simulink model "MotorControlLibNEWFixedP_FULL"  (R2020b)
settings: Solver=FixedStepDiscrete  StartTime=0.0  StopTime=100  FixedStep=Ts  RelTol=1e-3
values from neighbouring files (symbols this model uses):
  Ki_Iab_EMFobs = 1600.0    [MotorControl.sldd]
  Kp_Iab_EMFobs = 0.255    [MotorControl.sldd]
  p = 8/2    (= 4)    [MotorControlLibData.m]    (also in local_pmsm_torque_control_data.m = 8)
  Ts = 250.0e-06    (= 0.00025)    [MotorControlLibData.m]    (also in local_pmsm_torque_control_data.m = 5e-06)
undefined symbols (not defined in the file or in its folder): BrkPoints, CuttOffFreq_c, d_q_Voltage_Limiter_sat_neg, d_q_Voltage_Limiter_sat_pos, DiscIntNeverNeededParam, Down, dSoll, EMFobsLdGain, EMFobsRS, Ki_dAxis, Ki_qAxis, Kp_dAxis, Kp_qAxis, MaxBckEMFVol_sat_neg, MaxBckEMFVol_sat_pos, NumBits1, NumBits2, qSoll, Slope1, Slope2, TqToIqConst, TsIntern, Up
libraries: simulink x12, pid_lib x4, eePwmGenerator x3, simulink_extras x2
(part 1 of 2)
settings Model: DataDictionary=MotorControl.sldd  NumberOfSteps=50  Creator=unix  LastModifiedBy=unix
settings SolverCC: AutoInsertRateTranBlk=on
settings DebuggingCC: ArrayBoundsChecking=warning  SignalInfNanChecking=warning  SignalRangeChecking=warning  CheckMatrixSingularityMsg=warning  ParameterOverflowMsg=warning  ParameterUnderflowMsg=warning  ParameterPrecisionLossMsg=none  UnderSpecifiedDataTypeMsg=warning

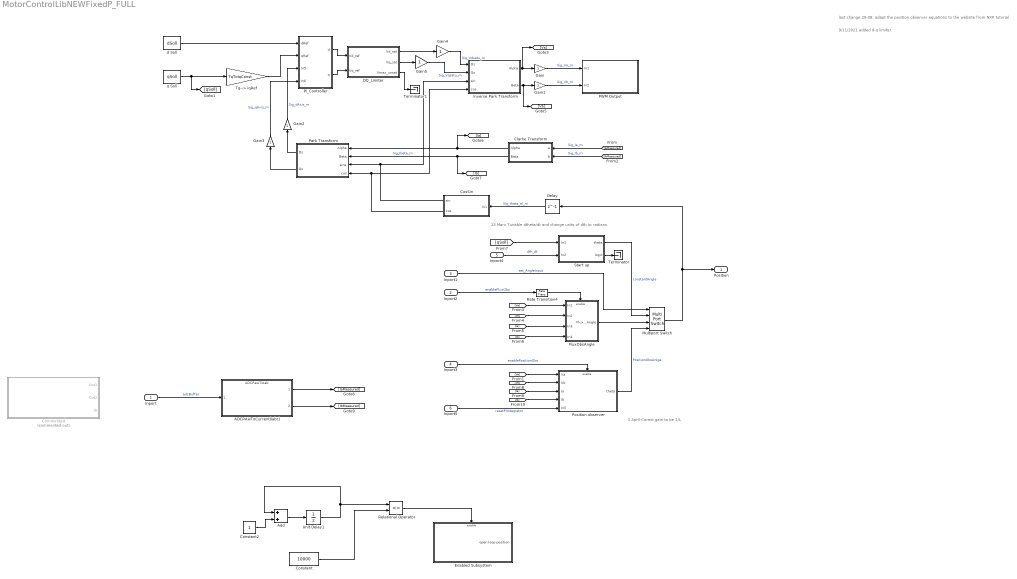
== system MotorControlLibNEWFixedP_FULL ==
  note: 3 April-Corect gain to be 1/L
  note: 9/11/2021 added d-q limiter.
  note: 23 Marz Tunable dtheta/dt and change units of dth to radians
  note: last change 29-08: adapt the position observer equations to the website from NXP tutorial
  Inport : Inport
  Inport2 : Inport  Port=2  OutDataTypeStr=boolean  SampleTime=5*Ts
      settings: AttributesFormatString=%<SampleTime>
  Inport1 : Inport  Port=3  OutDataTypeStr=uint8  SampleTime=5*Ts
      settings: AttributesFormatString=%<SampleTime>
  Inport3 : Inport  Port=4  OutDataTypeStr=boolean  SampleTime=5*Ts
      settings: AttributesFormatString=%<SampleTime>
  Inport4 : Inport  Port=5
  Inport5 : Inport  Port=6  OutDataTypeStr=boolean  SampleTime=5*Ts
      settings: AttributesFormatString=%<SampleTime>
  ADCRAwToCurrent(Iabc) : ModelReference  ModelNameDialog=ADCRawToIab  ModelReferenceVersion=3.2
  Add : Sum  OutDataTypeStr=uint16
  Clarke Transform : Subsystem  VariantControl=Variant2  mask(Clarke Transform){}
      mask help:
      | <p>Compute Clarke transformation on balanced 3-phase inputs into balanced 2-phase orthogonal outputs.
      | <br>
      | <br>
      | The block accepts two signals out of three phases, and outputs corresponding &alpha;-&beta; axis components, where phase-a axis is aligned with alpha axis.</p>
      mask Help: eval('mcb.internal.helpview(''clarketransform'')')
      mask Display: mcb.internal.drawIcons('Clarke',1);
  Commented : Subsystem  Commented=on
  Constant : Constant  Value=10000  OutDataTypeStr=uint16
  Constant2 : Constant  OutDataTypeStr=uint8
  CosSin : Subsystem
  DQ_Limiter : Subsystem  TreatAsAtomicUnit=on  SystemSampleTime=5*Ts  mask(DQ Limiter){Vmax=d_q_Voltage_Limiter_sat_pos}
      mask prompts: Vmax "D-Q saturation limit:"
      mask help:
      | Implement saturation on reference dq voltages, with respect to phase voltage peak limit.
      |
      | The block accepts reference values of d and q axis voltages, and outputs corresponding saturated values along with unsaturated peak value to initiate field weakening control.
      |
      | Enter the phase voltage peak limit in the dialog box to initiate saturation.
      settings: RTWFcnNameOpts=Use subsystem name
      mask Help: eval('mcb.internal.helpview(''dqlimiter'')')
  Delay : Delay  DelayLength=1  SampleTime=5*Ts
      settings: AttributesFormatString=%<SampleTime>
  Enabled Subsystem : Subsystem  TreatAsAtomicUnit=on
  FluxObsAngle : Subsystem
      settings: RTWFcnNameOpts=Use subsystem name
  Gain{,1..3} (4 alike) : Gain  OutDataTypeStr=Inherit: Same as input  ParamDataTypeStr=Inherit: Same as input
  Gain4 : Gain  OutDataTypeStr=Inherit: Inherit via back propagation
  Gain5 : Gain  OutDataTypeStr=Inherit: Inherit via back propagation
  Inverse Park Transform : Subsystem  SystemSampleTime=250*Ts  mask(Inverse Park Transform){AxisAlignment=D-axis}
      mask prompts: AxisAlignment "Alpha (phase-a) axis alignment:"
      mask help:
      | <p>Compute Inverse Park transformation on rotating reference frame inputs into stationary reference frame outputs.
      | <br><br>
      | The block accepts the following:
      | <ul>
      | <li>d-q axis components in rotating reference frame</li>
      | <li>Sine and cosine values of corresponding angle of transformation</li>
      | </ul>
      | The block outputs &alpha;-&beta; axis components in stationary reference frame.
      | <br><br>
      | D-axis alignment with alpha (phase-a) is popular in motor control theory while Q-axis alignment with alpha (phase-a) is more suitable for power conversion applications.</p>
      mask Help: eval('mcb.internal.helpview(''inverseparktransform'')')
      mask TypeOptions AxisAlignment: D-axis | Q-axis
  Multiport Switch : MultiPortSwitch  DataPortOrder=Zero-based contiguous  zeroidx=on
  PI_Controller : Subsystem  TreatAsAtomicUnit=on  SystemSampleTime=5*Ts
      settings: RTWFcnNameOpts=Use subsystem name
  PWM Output : Subsystem
  Park Transform : Subsystem  SystemSampleTime=250*Ts  mask(Park Transform){AxisAlignment=D-axis}
      mask prompts: AxisAlignment "Alpha (phase-a) axis alignment:"
      mask help:
      | <p>Compute Park transformation on stationary reference frame inputs into rotating reference frame outputs.
      | <br><br>
      | The block accepts the following:
      | <ul>
      |   <li>&alpha;-&beta; axis components in stationary reference frame</li>
      |   <li>Sine and cosine values of corresponding angle of transformation</li>
      | </ul>
      | The block outputs direct and quadrature axis components in rotating reference frame.
      | <br><br>
      | D-axis alignment with alpha (phase-a) is popular in motor control theory while Q-axis alignment with alpha (phase-a) is more suitable for power conversion applications.</p>
      mask Help: eval('mcb.internal.helpview(''parktransform'')')
      mask TypeOptions AxisAlignment: D-axis | Q-axis
      mask Display: mcb.internal.drawIcons('Park',1);
  Position observer : Subsystem
  Rate Transition4 : RateTransition
  Relational Operator : RelationalOperator  Operator=<=  OutDataTypeStr=boolean  RndMeth=Simplest
  Start up : Subsystem  TreatAsAtomicUnit=on  SystemSampleTime=5*Ts
  Terminator : Terminator
  Terminator1 : Terminator
  Tq--> iqRef : Gain  Gain=TqToIqConst  ParamDataTypeStr=Inherit: Inherit from 'Gain'  OutDataTypeStr=fixdt(1,16,2^-8,0)
  Unit Delay1 : UnitDelay  SampleTime=-1  HasFrameUpgradeWarning=on
  d Soll : Constant  Value=dSoll
  q Soll : Constant  Value=qSoll
  Position : Outport  SampleTime=250*Ts
  wires:
  ADCRAwToCurrent(Iabc)/2 -> [IbMeasured]
  Inport/1 -> ADCRAwToCurrent(Iabc)/1  "adcBuffer"
  ADCRAwToCurrent(Iabc)/1 -> [IaMeasured]
  Constant2/1 -> Add/2
  Unit Delay1/1 -> Relational Operator/1, Add/1
  Add/1 -> Unit Delay1/1
  Constant/1 -> Relational Operator/2
  Relational Operator/1 -> Enabled Subsystem/Enable
  Gain5/1 -> Inverse Park Transform/2(Qs)  "Sig_Vqsatu_m"
  PI_Controller/1(d) -> DQ_Limiter/1(Vd_ref)
  Inport3/1 -> Position observer/Enable  "enablePositionObs"
  Inverse Park Transform/1(Alpha) -> [Va], Gain/1
  Gain4/1 -> Inverse Park Transform/1(Ds)  "Sig_Vdsatu_m"
  Inport2/1 -> Rate Transition4/1  "enableFluxObs"
  DQ_Limiter/3(Vmax_unsat) -> Terminator1/1
  Park Transform/1(Ds) -> Gain2/1
  Start up/2(logic) -> Terminator/1
  Inport5/1 -> Position observer/5(In5)  "resetPIIntegrator"
  Gain2/1 -> PI_Controller/3(In5)  "Sig_dAxis_m"
  Gain1/1 -> PWM Output/2(In2)  "Sig_Vb_m"
  Gain3/1 -> PI_Controller/4(In6)  "Sig_qAxis_m"
  CosSin/1(sin) -> Inverse Park Transform/3(sin), Park Transform/3(sine)
  q Soll/1 -> [qSoll], Tq--> iqRef/1
  DQ_Limiter/1(Vd_sat) -> Gain4/1
  Inverse Park Transform/2(Beta) -> Gain1/1, [Vb]
  Clarke Transform/1(Alpha) -> [Ia], Park Transform/1(Alpha)
  Multiport Switch/1 -> Delay/1, Position/1
  d Soll/1 -> PI_Controller/1(dRef)
  [IaMeasured] -> Clarke Transform/1(a)  "Sig_Ia_m"
  [qSoll] -> Start up/1(In1)
  [Ib] -> FluxObsAngle/4(In4)
  [Vb] -> FluxObsAngle/2(In2)
  [Va] -> FluxObsAngle/1(In1)
  Gain/1 -> PWM Output/1(In1)  "Sig_Va_m"
  CosSin/2(cos) -> Inverse Park Transform/4(cos), Park Transform/4(cos)
  [Ia] -> FluxObsAngle/3(In3)
  Inport4/1 -> Start up/2(In2)  "dth_dt"
  PI_Controller/2(q) -> DQ_Limiter/2(Vq_ref)
  Delay/1 -> CosSin/1(In1)  "Sig_theta_el_m"
  Inport1/1 -> Multiport Switch/1  "set_AngleInput"
  FluxObsAngle/1(FluxObsAngle) -> Multiport Switch/3
  Park Transform/2(Qs) -> Gain3/1
  DQ_Limiter/2(Vq_sat) -> Gain5/1
  Rate Transition4/1 -> FluxObsAngle/Enable
  [IbMeasured] -> Clarke Transform/2(b)  "Sig_Ib_m"
  Clarke Transform/2(Beta) -> [Ib], Park Transform/2(Beta)  "Sig_Ibeta_m"
  Tq--> iqRef/1 -> PI_Controller/2(qRef)
  Position observer/1(theta) -> Multiport Switch/4  "PositionObsAnlge"
  Start up/1(theta) -> Multiport Switch/2  "constantAngle"
  [Va] -> Position observer/1(Va)
  [Vb] -> Position observer/2(Vb)
  [Ia] -> Position observer/3(Ia)
  [Ib] -> Position observer/4(Ib)

== system MotorControlLibNEWFixedP_FULL/Clarke Transform ==
  a : Inport
  b : Inport  Port=2
  Data Type Duplicate : DataTypeDuplicate
  a_plus_2b : Sum  Inputs=+++  RndMeth=Simplest  OutDataTypeStr=Inherit: Same as first input
  one_by_sqrt3 : Gain  Gain=1/sqrt(3)  RndMeth=Simplest  OutDataTypeStr=Inherit: Same as input
  Alpha : Outport  VectorParamsAs1DForOutWhenUnconnected=off
  Beta : Outport  Port=2  VectorParamsAs1DForOutWhenUnconnected=off
  wires:
  a/1 -> a_plus_2b/1, Alpha/1, Data Type Duplicate/1
  one_by_sqrt3/1 -> Beta/1
  a_plus_2b/1 -> one_by_sqrt3/1
  b/1 -> a_plus_2b/2, a_plus_2b/3, Data Type Duplicate/2

== system MotorControlLibNEWFixedP_FULL/Commented ==
  Digital Clock : DigitalClock  Commented=on  SampleTime=Ts
  Function-Call Clock_50us : simulink/Ports & Subsystems/Function-Call Generator  Commented=on  sample_time=5e-5  numberOfIterations=1  DisallowWideOutput=off
  Function-Call Clock_50us1 : simulink/Ports & Subsystems/Function-Call Generator  Commented=on  sample_time=Ts  numberOfIterations=1  DisallowWideOutput=off
  Function-Call Split : FunctionCallSplit  Commented=on  IconShape=distinctive  NumOutputPorts=3  OutputPortLayout=default
  Goto1 : Goto  Commented=on  GotoTag=Task100us_2
  Goto2 : Goto  Commented=on  GotoTag=Task100us_1
  Goto4 : Goto  Commented=on  GotoTag=Task1ms_1
  Rate Transition8 : RateTransition  Commented=on
  Subsystem : Subsystem  Commented=on
  Task Scheduler : Stateflow chart  Commented=on  TreatAsAtomicUnit=on
  Out1 : Outport
  Out2 : Outport  Port=2
  dt : Outport  Port=3
  wires:
  Task Scheduler/2(Task_100us_2()) -> Goto1/1
  Function-Call Clock_50us/1 -> Task Scheduler/Trigger
  Digital Clock/1 -> Rate Transition8/1
  Rate Transition8/1 -> Subsystem/1(Clock)
  Function-Call Clock_50us1/1 -> Function-Call Split/1
  Function-Call Split/3 -> Subsystem/Trigger
  Subsystem/1(dt) -> dt/1
  Function-Call Split/2 -> Out2/1
  Function-Call Split/1 -> Out1/1
  Task Scheduler/1(Task_100us_1()) -> Goto2/1
  Task Scheduler/3(Task_1ms_1()) -> Goto4/1

== system MotorControlLibNEWFixedP_FULL/CosSin ==
  In1 : Inport
  Data Type Conversion1 : DataTypeConversion
  Sine-Cosine Lookup : Subsystem  mask(Sine-Cosine Lookup){AngleInput=Radians, N_points=512}
      mask prompts: AngleInput "Theta units:"; N_points "Number of data points for lookup table:"
      mask help:
      | Implement sine and cosine functions using a lookup table approach for optimized performance on target hardware.
      |
      | The block accepts input angle in different units and outputs corresponding sine and cosine values.
      mask init:
      | % dlgSett = mct.internal.SinCosCb(gcbh);
      | this = get_param(gcbh,'Object');
      | 
      | points = eval(this.N_points);
      | 
      | dlgSett.points = 125*floor(points/125);
      | 
      | dlgSett.Offset = uint16(dlgSett.points/5);
      | 
      | dlgSett.N_points = 4*dlgSett.Offset;
      | N_points = dlgSett.N_points;
      | 
      | theta = linspace(0,2*pi,N_points+1);
      | dlgSett.size = 5*dlgSett.Offset+2;
      | dlgSett.sin_table = zeros(1,dlgSett.size);
      | dlgSett.sin_table(1:N_points+1) = sin(theta);
      | dlgSett.sin_table(N_points+2:dlgSett.size) = dlgSett.sin_table(2:0.25*N_points+2);
      | 
      | dlgSett.N_points = double(dlgSett.N_points);
      | dlgSett.index_gain = dlgSett.N_points;
      | dlgSett.UpperSatLimit = 1;
      | 
      | switch AngleInput
      |     case 1
      |         dlgSett.UpperSatLimit = 1;
      |     case 2
      |         dlgSett.UpperSatLimit = 2*pi;
      |     case 3
      |         dlgSett.UpperSatLimit = 360;
      |     otherwise
      | end
      mask Help: eval('mcb.internal.helpview(''sinecosinelookup'')')
      mask TypeOptions AngleInput: Per-unit | Radians | Degrees
      mask Display: mcb.internal.drawIcons('Sin-Cos',1);
  sin : Outport
  cos : Outport  Port=2
  wires:
  Sine-Cosine Lookup/2(cos) -> cos/1
  In1/1 -> Data Type Conversion1/1
  Sine-Cosine Lookup/1(sin) -> sin/1
  Data Type Conversion1/1 -> Sine-Cosine Lookup/1(Theta)

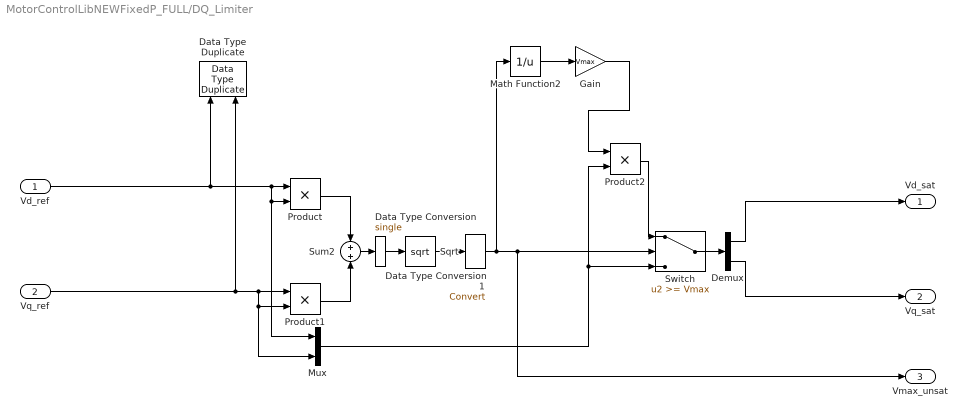
== system MotorControlLibNEWFixedP_FULL/DQ_Limiter ==
  Vd_ref : Inport
  Vq_ref : Inport  Port=2
  Data Type Duplicate : DataTypeDuplicate
  Data Type Conversion : DataTypeConversion  OutDataTypeStr=single
  Data Type Conversion1 : DataTypeConversion
  Demux : Demux  Outputs=2
  Gain : Gain  Gain=Vmax  OutDataTypeStr=Inherit: Same as input
  Math Function2 : Math  Operator=reciprocal  SignedPower=on  RndMeth=Simplest
  Mux : Mux  Inputs=2
  Product : Product  RndMeth=Simplest  OutDataTypeStr=Inherit: Same as first input
  Product1 : Product  RndMeth=Simplest  OutDataTypeStr=Inherit: Same as first input
  Product2 : Product  OutDataTypeStr=Inherit: Same as first input
  Sqrt : Sqrt  IntermediateResultsDataTypeStr=Inherit: Inherit from input  SaturateOnIntegerOverflow=on
  Sum2 : Sum  OutDataTypeStr=Inherit: Same as first input
  Switch : Switch  Threshold=Vmax  ZeroCross=off
  Vd_sat : Outport  VectorParamsAs1DForOutWhenUnconnected=off
  Vq_sat : Outport  Port=2  VectorParamsAs1DForOutWhenUnconnected=off
  Vmax_unsat : Outport  Port=3  VectorParamsAs1DForOutWhenUnconnected=off
  wires:
  Vd_ref/1 -> Data Type Duplicate/1, Product/1, Product/2, Mux/1
  Demux/1 -> Vd_sat/1
  Product1/1 -> Sum2/2
  Product/1 -> Sum2/1
  Sum2/1 -> Data Type Conversion/1
  Math Function2/1 -> Gain/1
  Mux/1 -> Product2/2, Switch/3
  Product2/1 -> Switch/1
  Switch/1 -> Demux/1
  Demux/2 -> Vq_sat/1
  Sqrt/1 -> Data Type Conversion1/1
  Gain/1 -> Product2/1
  Vq_ref/1 -> Data Type Duplicate/2, Product1/1, Product1/2, Mux/2
  Data Type Conversion1/1 -> Vmax_unsat/1, Switch/2, Math Function2/1
  Data Type Conversion/1 -> Sqrt/1

== system MotorControlLibNEWFixedP_FULL/Enabled Subsystem ==
  Enable : EnablePort  StatesWhenEnabling=reset
  Constant : Constant  Value=66.67  OutDataTypeStr=fixdt(1,16,2^-7,0)
  Constant1 : Constant  Value=2*pi  OutDataTypeStr=fixdt(1,16,2^-7,0)
  Discrete-Time Integrator : DiscreteIntegrator  ExternalReset=rising  SampleTime=-1  OutDataTypeStr=fixdt(1,16,2^-8,0)  SaturateOnIntegerOverflow=on  ICPrevOutput=DiscIntNeverNeededParam  ICPrevScaledInput=DiscIntNeverNeededParam
  Gain4 : Gain  Gain=2*pi  ParamDataTypeStr=fixdt(1,16,2^-7,0)  OutDataTypeStr=fixdt(1,16,2^-5,0)
  Gain5 : Gain  Gain=(30/pi)/p
  Relational Operator : RelationalOperator  OutDataTypeStr=boolean  RndMeth=Simplest
  Scope : Scope  NumInputPorts=2
  Unit Delay : UnitDelay  SampleTime=-1  HasFrameUpgradeWarning=on
  open loop position : Outport
  wires:
  Constant/1 -> Gain4/1
  Discrete-Time Integrator/1 -> open loop position/1, Scope/1, Relational Operator/1
  Gain4/1 -> Gain5/1, Discrete-Time Integrator/1
  Unit Delay/1 -> Discrete-Time Integrator/2
  Relational Operator/1 -> Unit Delay/1
  Gain5/1 -> Scope/2
  Constant1/1 -> Relational Operator/2

== system MotorControlLibNEWFixedP_FULL/FluxObsAngle ==
  In1 : Inport
  In2 : Inport  Port=2
  In3 : Inport  Port=3
  In4 : Inport  Port=4
  Enable : EnablePort
  Flux Observer : Subsystem  TreatAsAtomicUnit=on  SystemSampleTime=5*Ts  mask(Flux Observer){BlockInputUnit=SI unit, PerUnitVoltage=13.86, PerUnitCurrent=19.3, PositionSelect=on, FluxSelect=off, TorqueSelect=off, PolePairs=4, StatorResistance=EMFobsRS, StatorDAxisInductance=EMFobsLdGain, BlockSampleTime=5*Ts, PositionUnit=Radians, PositionDatatype=fixdt(1,16,2^-8,0), FluxUnit=Weber, PerUnitFlux=0.1, FluxDatatype=single, TorqueUnit=Nm, PerUnitTorque=100, TorqueDatatype=single}
      mask prompts: BlockInputUnit "Input units:"; PerUnitVoltage "Per unit reference voltage (V):"; PerUnitCurrent "Per unit reference current (A):"; PositionSelect "Position"; FluxSelect "Flux"; TorqueSelect "Torque"; PolePairs "Pole pairs:"; StatorResistance "Stator resistance (ohm):"; StatorDAxisInductance "Stator d-axis inductance (H):"; BlockSampleTime "Block sample time (S):"; PositionUnit "Position unit:"; PositionDatatype "Position datatype:"; FluxUnit "Flux unit:"; PerUnitFlux "Per unit flux (Wb):"; FluxDatatype "Flux datatype:"; TorqueUnit "Torque unit:"; PerUnitTorque "Per unit torque (Nm):"; TorqueDatatype "Torque datatype:"
      mask help:
      | <p>Compute &#952;<sub>e</sub> (electrical position), &#936; (magnetic flux), and T<sub>e</sub> (electrical torque) of a PMSM from the measured voltage and current in the stationary reference frame.
      | <br><br>
      | Use the Input units parameter to select the input unit of the block.
      | <br><br>
      | Use the Per unit reference voltage parameter to enter the amplitude of line-to-neutral voltage used as a reference. Use the Per unit reference current parameter to enter the amplitude of line current used as a reference.</P>
      mask init:
      | %mcb.internal.FOCb('MaskInitFcn', gcbh);
      mask Help: eval('mcb.internal.helpview(''fluxobserver'')')
      mask TypeOptions BlockInputUnit: SI unit | Per-unit
      mask Callback BlockInputUnit: mcb.internal.FOCb('MaskDisplay', gcbh);
      mask Callback PositionSelect: mcb.internal.FOCb('MaskDisplay', gcbh);
      mask Callback FluxSelect: mcb.internal.FOCb('MaskDisplay', gcbh);
      mask Callback TorqueSelect: mcb.internal.FOCb('MaskDisplay', gcbh);
      mask TypeOptions PositionUnit: Radians | Degrees | Per-unit
      mask TypeOptions FluxUnit: Weber | Per-unit
      mask Callback FluxUnit: mcb.internal.FOCb('MaskDisplay', gcbh);
      mask TypeOptions TorqueUnit: Nm | Per-unit
      mask Callback TorqueUnit: mcb.internal.FOCb('MaskDisplay', gcbh);
      mask DialogControl Container4 Prompt: Motor Parameters
      mask DialogControl Container7 Prompt: Block Output
      mask DialogControl Container8 Prompt: Datatypes
      mask Display:
      | color('black');
      | port_label('input',1, 'V_{\alpha}', 'interpreter', 'tex');
      | port_label('input',2, 'V_{\beta}', 'interpreter', 'tex');
      | port_label('input',3, 'I_{\alpha}', 'interpreter', 'tex');
      | port_label('input',4, 'I_{\beta}', 'interpreter', 'tex');
      | port_label('input',5, 'Rst', 'interpreter', 'tex');
      | port_label('output',1, '\theta_{e}', 'interpreter', 'tex');
      | %No Flux;
      | %No Torque;
      | fprintf('Flux\nObserver');
  Ground : Ground
  FluxObsAngle : Outport
  wires:
  In1/1 -> Flux Observer/1(Valpha)
  Ground/1 -> Flux Observer/5(Reset)
  In4/1 -> Flux Observer/4(Ibeta)
  In2/1 -> Flux Observer/2(Vbeta)
  In3/1 -> Flux Observer/3(Ialpha)
  Flux Observer/1(Position) -> FluxObsAngle/1  "FluxObsAngle"

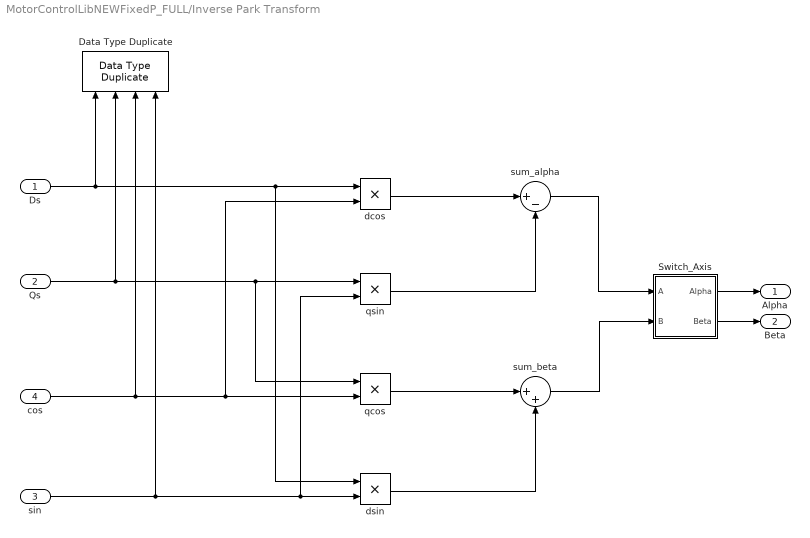
== system MotorControlLibNEWFixedP_FULL/Inverse Park Transform ==
  Ds : Inport
  Qs : Inport  Port=2
  sin : Inport  Port=3
  cos : Inport  Port=4
  Data Type Duplicate : DataTypeDuplicate  NumInputPorts=4
  Switch_Axis : Subsystem
  dcos : Product  RndMeth=Simplest  OutDataTypeStr=Inherit: Same as first input
  dsin : Product  RndMeth=Simplest  OutDataTypeStr=Inherit: Same as first input
  qcos : Product  RndMeth=Simplest  OutDataTypeStr=Inherit: Same as first input
  qsin : Product  RndMeth=Simplest  OutDataTypeStr=Inherit: Same as first input
  sum_alpha : Sum  Inputs=|+-  RndMeth=Simplest  OutDataTypeStr=Inherit: Same as first input
  sum_beta : Sum  Inputs=|++  RndMeth=Simplest  OutDataTypeStr=Inherit: Same as first input
  Alpha : Outport  VectorParamsAs1DForOutWhenUnconnected=off
  Beta : Outport  Port=2  VectorParamsAs1DForOutWhenUnconnected=off
  wires:
  Switch_Axis/2(Beta) -> Beta/1
  Switch_Axis/1(Alpha) -> Alpha/1
  sum_beta/1 -> Switch_Axis/2(B)
  sum_alpha/1 -> Switch_Axis/1(A)
  sin/1 -> dsin/2, qsin/2, Data Type Duplicate/4
  cos/1 -> qcos/2, dcos/2, Data Type Duplicate/3
  dsin/1 -> sum_beta/2
  Qs/1 -> qsin/1, qcos/1, Data Type Duplicate/2
  dcos/1 -> sum_alpha/1
  qcos/1 -> sum_beta/1
  qsin/1 -> sum_alpha/2
  Ds/1 -> dcos/1, dsin/1, Data Type Duplicate/1

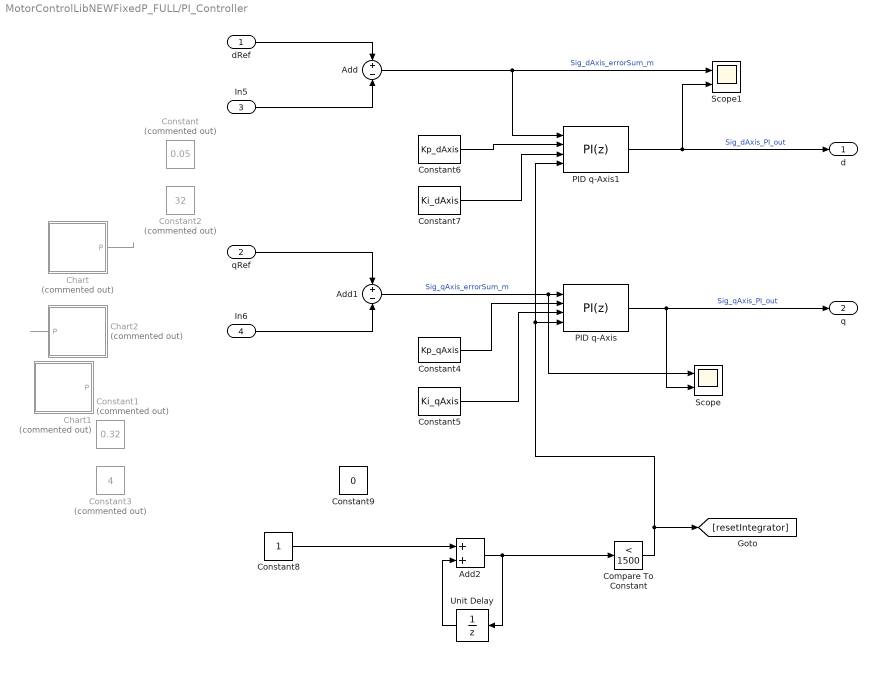
== system MotorControlLibNEWFixedP_FULL/PI_Controller ==
  dRef : Inport
  qRef : Inport  Port=2
  In5 : Inport  Port=3
  In6 : Inport  Port=4
  Add : Sum  Inputs=+|-
  Add1 : Sum  Inputs=+|-
  Add2 : Sum
  Chart : Stateflow chart  Commented=on  TreatAsAtomicUnit=on  SystemSampleTime=1000*Ts
  Chart1 : Stateflow chart  Commented=on  TreatAsAtomicUnit=on  SystemSampleTime=2000*Ts
  Chart2 : Stateflow chart  Commented=on  TreatAsAtomicUnit=on  SystemSampleTime=100000*Ts
  Compare To Constant : simulink/Logic and Bit Operations/Compare To Constant  relop=<  const=1500  OutDataTypeStr=boolean
  Constant : Constant  Commented=on  Value=0.05  OutDataTypeStr=fixdt(1,16,2^-7,0)
  Constant1 : Constant  Commented=on  Value=0.32  OutDataTypeStr=fixdt(1,8,2^-7,0)
  Constant2 : Constant  Commented=on  Value=32  OutDataTypeStr=fixdt(1,8,2^-1,0)
  Constant3 : Constant  Commented=on  Value=4  OutDataTypeStr=fixdt(1,8,2^-1,0)
  Constant4 : Constant  Value=Kp_qAxis
  Constant5 : Constant  Value=Ki_qAxis
  Constant6 : Constant  Value=Kp_dAxis
  Constant7 : Constant  Value=Ki_dAxis
  Constant8 : Constant
  Constant9 : Constant  Value=0  OutDataTypeStr=boolean
  PID q-Axis : pid_lib/PID Controller  Controller=PI  Form=Parallel  TimeDomain=Discrete-time  UseExternalTs=off  SampleTime=-1  IntegratorMethod=Forward Euler  FilterMethod=Forward Euler  ControllerParametersSource=external  P=0  I=0  D=0  UseFilter=on  N=100  TunerSelectOption=Transfer Function Based (PID Tuner App)  InitialConditionSource=internal  InitialConditionForIntegrator=0  InitialConditionForFilter=0  DifferentiatorICPrevScaledInput=0  ExternalReset=level  TrackingMode=off  Kt=1  LimitOutput=on  SatLimitsSource=internal  UpperSaturationLimit=d_q_Voltage_Limiter_sat_pos  LowerSaturationLimit=d_q_Voltage_Limiter_sat_neg  LinearizeAsGain=off  AntiWindupMode=clamping  Kb=10  PGainOutDataTypeStr=fixdt(1,16,2^-8,0)  PProdOutDataTypeStr=fixdt(1,16,2^-8,0)  POutMin=[]  POutMax=[]  IGainOutDataTypeStr=fixdt(1,16,2^-8,0)  IProdOutDataTypeStr=fixdt(1,16,2^-8,0)  IOutMin=[]  IOutMax=[]  DOutMin=[]  DOutMax=[]  NOutMin=[]  NOutMax=[]  SumOutDataTypeStr=fixdt(1,16,2^-8,0)  SumOutMin=[]  SumOutMax=[]  SaturationOutMin=[]  SaturationOutMax=[]  PParamMin=[]  PParamMax=[]  IParamMin=[]  IParamMax=[]  DParamMin=[]  DParamMax=[]  NParamMin=[]  NParamMax=[]  KbParamMin=[]  KbParamMax=[]  KtParamMin=[]  KtParamMax=[]  KbOutMin=[]  KbOutMax=[]  KtOutMin=[]  KtOutMax=[]  IntegratorOutDataTypeStr=fixdt(1,16,2^-8,0)  IntegratorOutMin=[]  IntegratorOutMax=[]  FilterOutMin=[]  FilterOutMax=[]  SumI1OutMin=[]  SumI1OutMax=[]  SumI2OutMin=[]  SumI2OutMax=[]  SumI3OutMin=[]  SumI3OutMax=[]  SumI4OutMin=[]  SumI4OutMax=[]  SumDOutMin=[]  SumDOutMax=[]  SumAccumDataTypeStr=fixdt(1,16,2^-8,0)  DifferentiatorOutMin=[]  DifferentiatorOutMax=[]  FilterDiffOutCoefMin=[]  FilterDiffOutCoefMax=[]  ReciprocalOutMin=[]  ReciprocalOutMax=[]  SumDenOutMin=[]  SumDenOutMax=[]  SumNumOutMin=[]  SumNumOutMax=[]  DivideOutMin=[]  DivideOutMax=[]  UdiffTsProdOutMin=[]  UdiffTsProdOutMax=[]  NTsProdOutMin=[]  NTsProdOutMax=[]  UintegralTsProdOutMin=[]  UintegralTsProdOutMax=[]  UngainTsProdOutMin=[]  UngainTsProdOutMax=[]  IntegratorContinuousStateAttributes=''  IntegratorStateMustResolveToSignalObject=off  IntegratorRTWStateStorageClass=Auto  FilterContinuousStateAttributes=''  FilterStateMustResolveToSignalObject=off  FilterRTWStateStorageClass=Auto  ParallelPVariant=ExternalParameters  IdealPVariant=Disabled  IVariant=ExternalParameters  DVariant=Disabled  IntegratorVariant=Discrete  SatVariant=Enabled  AWVariant=DiscClampingParallel  PCopyVariant=Disabled  TRVariant=Disabled  FdbkBlocksVariant=Forward  IdealPFdbkVariant=Disabled  SatFdbkVariant=Disabled  DerivativeFilterVariant=Disabled  NVariant=Disabled  NCopyVariant=Disabled_SignalSpec  FilterICVariant=Disabled  IntegratorICVariant=InternalICs  ExternalResetVariant=ExternalReset  TRSumVariant=Passthrough  SumFdbkVariant=Disabled  SumVariant=Sum_PI  TsampFilterVariant=InternalTs  TsampNgainVariant=Passthrough  TsampIntegralVariant=Passthrough  ExternalSaturationOutDataTypeStr=Inherit: Same as second input
  PID q-Axis1 : pid_lib/PID Controller  Controller=PI  Form=Parallel  TimeDomain=Discrete-time  UseExternalTs=off  SampleTime=-1  IntegratorMethod=Forward Euler  FilterMethod=Forward Euler  ControllerParametersSource=external  P=0  I=0  D=0  UseFilter=on  N=100  TunerSelectOption=Transfer Function Based (PID Tuner App)  ZeroCross=off  InitialConditionSource=internal  InitialConditionForIntegrator=0  InitialConditionForFilter=0  DifferentiatorICPrevScaledInput=0  ExternalReset=level  TrackingMode=off  Kt=1  LimitOutput=on  SatLimitsSource=internal  UpperSaturationLimit=d_q_Voltage_Limiter_sat_pos  LowerSaturationLimit=d_q_Voltage_Limiter_sat_neg  LinearizeAsGain=off  AntiWindupMode=clamping  Kb=10  PGainOutDataTypeStr=fixdt(1,16,2^-8,0)  PProdOutDataTypeStr=fixdt(1,16,2^-8,0)  POutMin=[]  POutMax=[]  IGainOutDataTypeStr=fixdt(1,16,2^-8,0)  IProdOutDataTypeStr=fixdt(1,16,2^-8,0)  IOutMin=[]  IOutMax=[]  DOutMin=[]  DOutMax=[]  NOutMin=[]  NOutMax=[]  SumOutDataTypeStr=fixdt(1,16,2^-8,0)  SumOutMin=[]  SumOutMax=[]  SaturationOutMin=[]  SaturationOutMax=[]  PParamMin=[]  PParamMax=[]  IParamMin=[]  IParamMax=[]  DParamMin=[]  DParamMax=[]  NParamMin=[]  NParamMax=[]  KbParamMin=[]  KbParamMax=[]  KtParamMin=[]  KtParamMax=[]  KbOutMin=[]  KbOutMax=[]  KtOutMin=[]  KtOutMax=[]  IntegratorOutDataTypeStr=fixdt(1,16,2^-8,0)  IntegratorOutMin=[]  IntegratorOutMax=[]  FilterOutMin=[]  FilterOutMax=[]  SumI1OutMin=[]  SumI1OutMax=[]  SumI2OutMin=[]  SumI2OutMax=[]  SumI3OutMin=[]  SumI3OutMax=[]  SumI4OutMin=[]  SumI4OutMax=[]  SumDOutMin=[]  SumDOutMax=[]  SumAccumDataTypeStr=fixdt(1,16,2^-8,0)  DifferentiatorOutMin=[]  DifferentiatorOutMax=[]  FilterDiffOutCoefMin=[]  FilterDiffOutCoefMax=[]  ReciprocalOutMin=[]  ReciprocalOutMax=[]  SumDenOutMin=[]  SumDenOutMax=[]  SumNumOutMin=[]  SumNumOutMax=[]  DivideOutMin=[]  DivideOutMax=[]  UdiffTsProdOutMin=[]  UdiffTsProdOutMax=[]  NTsProdOutMin=[]  NTsProdOutMax=[]  UintegralTsProdOutMin=[]  UintegralTsProdOutMax=[]  UngainTsProdOutMin=[]  UngainTsProdOutMax=[]  IntegratorContinuousStateAttributes=''  IntegratorStateMustResolveToSignalObject=off  IntegratorRTWStateStorageClass=Auto  FilterContinuousStateAttributes=''  FilterStateMustResolveToSignalObject=off  FilterRTWStateStorageClass=Auto  ParallelPVariant=ExternalParameters  IdealPVariant=Disabled  IVariant=ExternalParameters  DVariant=Disabled  IntegratorVariant=Discrete  SatVariant=Enabled  AWVariant=DiscClampingParallel  PCopyVariant=Disabled  TRVariant=Disabled  FdbkBlocksVariant=Forward  IdealPFdbkVariant=Disabled  SatFdbkVariant=Disabled  DerivativeFilterVariant=Disabled  NVariant=Disabled  NCopyVariant=Disabled_SignalSpec  FilterICVariant=Disabled  IntegratorICVariant=InternalICs  ExternalResetVariant=ExternalReset  TRSumVariant=Passthrough  SumFdbkVariant=Disabled  SumVariant=Sum_PI  TsampFilterVariant=InternalTs  TsampNgainVariant=Passthrough  TsampIntegralVariant=Passthrough  ExternalSaturationOutDataTypeStr=Inherit: Same as second input
  Scope : Scope  NumInputPorts=2
  Scope1 : Scope  NumInputPorts=2
  Unit Delay : UnitDelay  SampleTime=-1  HasFrameUpgradeWarning=on
  d : Outport
  q : Outport  Port=2
  wires:
  dRef/1 -> Add/1
  qRef/1 -> Add1/1
  In6/1 -> Add1/2
  PID q-Axis/1 -> Scope/2, q/1  "Sig_qAxis_PI_out"
  PID q-Axis1/1 -> Scope1/2, d/1  "Sig_dAxis_PI_out"
  In5/1 -> Add/2
  Add1/1 -> Scope/1, PID q-Axis/1  "Sig_qAxis_errorSum_m"
  Chart/1(P) -> ?
  Chart2/1(P) -> ?
  Constant5/1 -> PID q-Axis/3
  Constant4/1 -> PID q-Axis/2
  Add/1 -> Scope1/1, PID q-Axis1/1  "Sig_dAxis_errorSum_m"
  Constant6/1 -> PID q-Axis1/2
  Constant7/1 -> PID q-Axis1/3
  Constant8/1 -> Add2/1
  Add2/1 -> Unit Delay/1, Compare To Constant/1
  Unit Delay/1 -> Add2/2
  Compare To Constant/1 -> [resetIntegrator], PID q-Axis1/4, PID q-Axis/4

== system MotorControlLibNEWFixedP_FULL/PWM Output ==
  In1 : Inport
  In2 : Inport  Port=2
  1-D Lookup Table : Lookup_n-D  NumberOfTableDimensions=1  BreakpointsForDimension1=BrkPoints  Table=[0 500 1000]  ExtrapMethod=Clip  InternalRulePriority=Speed  OutDataTypeStr=uint16  RndMeth=Simplest  SaturateOnIntegerOverflow=on  InputSameDT=on
  1-D Lookup Table1 : Lookup_n-D  NumberOfTableDimensions=1  BreakpointsForDimension1=BrkPoints  Table=[0 500 1000]  ExtrapMethod=Clip  InternalRulePriority=Speed  OutDataTypeStr=uint16  RndMeth=Simplest  SaturateOnIntegerOverflow=on  InputSameDT=on
  1-D Lookup Table2 : Lookup_n-D  NumberOfTableDimensions=1  BreakpointsForDimension1=BrkPoints  Table=[0 500 1000]  ExtrapMethod=Clip  InternalRulePriority=Speed  OutDataTypeStr=uint16  RndMeth=Simplest  SaturateOnIntegerOverflow=on  InputSameDT=on
  Data Type Conversion : DataTypeConversion
  Data Type Conversion1 : DataTypeConversion
  Data Type Conversion2 : DataTypeConversion
  Inverse Clarke Transform : Subsystem  mask(Inverse Clarke Transform){}
      mask help:
      | <p>Compute Inverse Clarke transformation on balanced 2-phase orthogonal inputs into balanced 3-phase outputs.
      | <br><br>
      | The block accepts &alpha;-&beta; axis components and outputs corresponding 3-phase outputs, where phase-a axis is aligned with &alpha;-axis.</p>
      mask Help: eval('mcb.internal.helpview(''inverseclarketransform'')')
      mask Display: mcb.internal.drawIcons('invClarke',1);
  PWM Generator : eePwmGenerator/PWM Generator  Commented=on  CarrCount=Up-Down  Tper=10*Ts  Ts=Ts
  PWM Generator1 : eePwmGenerator/PWM Generator  Commented=on  CarrCount=Up-Down  Tper=10*Ts  Ts=Ts
  PWM Generator2 : eePwmGenerator/PWM Generator  Commented=on  CarrCount=Up-Down  Tper=10*Ts  Ts=Ts
  Scope : Scope  Commented=on  NumInputPorts=3
  wires:
  In2/1 -> Inverse Clarke Transform/2(In2)
  In1/1 -> Inverse Clarke Transform/1(In1)
  Inverse Clarke Transform/1(a) -> 1-D Lookup Table/1
  1-D Lookup Table/1 -> Data Type Conversion/1
  Inverse Clarke Transform/2(b) -> 1-D Lookup Table1/1
  Inverse Clarke Transform/3(c) -> 1-D Lookup Table2/1
  PWM Generator/1 -> Scope/1
  1-D Lookup Table2/1 -> Data Type Conversion2/1
  1-D Lookup Table1/1 -> Data Type Conversion1/1
  PWM Generator1/1 -> Scope/2
  PWM Generator2/1 -> Scope/3
  Data Type Conversion/1 -> PWM Generator/1  "PWM_A_DT"
  Data Type Conversion1/1 -> PWM Generator1/1  "PWM_B_DT"
  Data Type Conversion2/1 -> PWM Generator2/1  "PWM_C_DT"

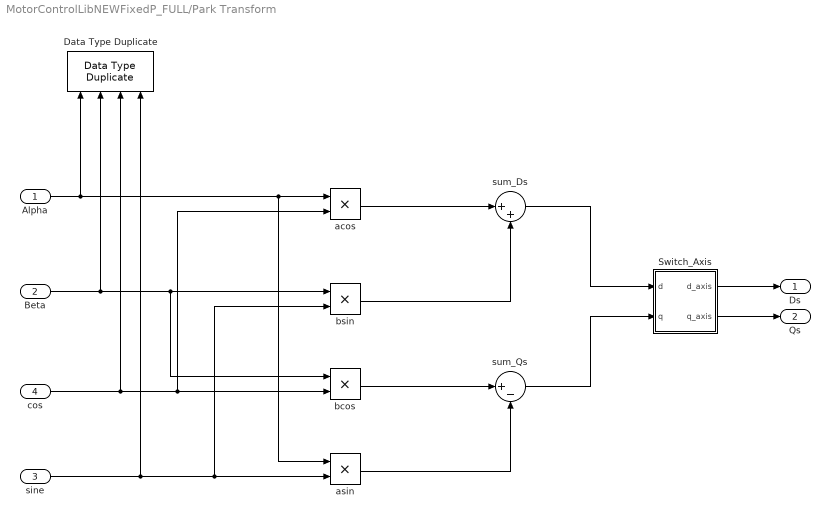
== system MotorControlLibNEWFixedP_FULL/Park Transform ==
  Alpha : Inport
  Beta : Inport  Port=2
  sine : Inport  Port=3
  cos : Inport  Port=4
  Data Type Duplicate : DataTypeDuplicate  NumInputPorts=4
  Switch_Axis : Subsystem
  acos : Product  RndMeth=Simplest  OutDataTypeStr=Inherit: Same as first input
  asin : Product  RndMeth=Simplest  OutDataTypeStr=Inherit: Same as first input
  bcos : Product  OutDataTypeStr=Inherit: Inherit via back propagation  RndMeth=Simplest
  bsin : Product  OutDataTypeStr=Inherit: Inherit via back propagation  RndMeth=Simplest
  sum_Ds : Sum  Inputs=|++  RndMeth=Simplest  OutDataTypeStr=Inherit: Same as first input
  sum_Qs : Sum  Inputs=|+-  RndMeth=Simplest  OutDataTypeStr=Inherit: Same as first input
  Ds : Outport  VectorParamsAs1DForOutWhenUnconnected=off
  Qs : Outport  Port=2  VectorParamsAs1DForOutWhenUnconnected=off
  wires:
  Beta/1 -> Data Type Duplicate/2, bcos/1, bsin/1
  Switch_Axis/1(d_axis) -> Ds/1
  Switch_Axis/2(q_axis) -> Qs/1
  sum_Ds/1 -> Switch_Axis/1(d)
  sum_Qs/1 -> Switch_Axis/2(q)
  cos/1 -> Data Type Duplicate/3, bcos/2, acos/2
  asin/1 -> sum_Qs/2
  bcos/1 -> sum_Qs/1
  bsin/1 -> sum_Ds/2
  acos/1 -> sum_Ds/1
  Alpha/1 -> Data Type Duplicate/1, acos/1, asin/1
  sine/1 -> bsin/2, asin/2, Data Type Duplicate/4

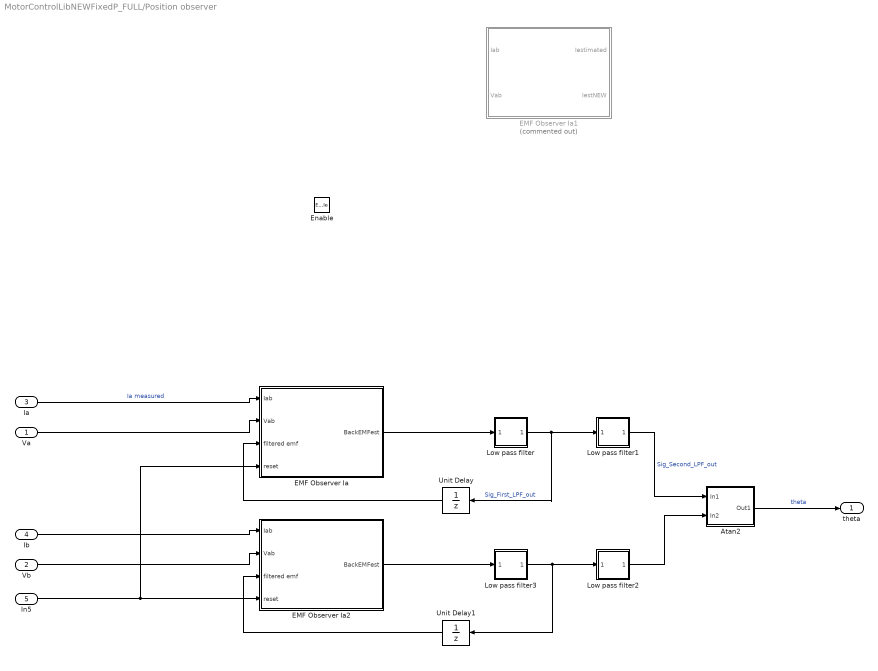
== system MotorControlLibNEWFixedP_FULL/Position observer ==
  Va : Inport
  Vb : Inport  Port=2
  Ia : Inport  Port=3
  Ib : Inport  Port=4
  In5 : Inport  Port=5
  Enable : EnablePort  StatesWhenEnabling=reset
  Atan2 : Subsystem
  EMF Observer Ia : Subsystem  mask{Rs=EMFobsRS, Ld=EMFobsLdGain, P=Kp_Iab_EMFobs, I=Ki_Iab_EMFobs}
      mask prompts: Rs "Resistance"; Ld "Inductance"; P "Simulink:masks:ProportionalP_MP"; I "Simulink:masks:IntegralI_MP"
      mask TypeOptions Rs: DC Motor Model/Resistance/Gain
      mask TypeOptions Ld: DC Motor Model/Inductance/Gain
      mask TypeOptions P: PID Controller/P
      mask TypeOptions I: PID Controller/I
      mask DialogControl Container6 Prompt: PI Controller
      mask DialogControl P Prompt: Proportional (P):
      mask DialogControl I Prompt: Integral (I):
  EMF Observer Ia1 : Subsystem  Commented=on  mask{Rs=EMFobsRS, Ld=EMFobsLdGain, P=Kp_Iab_EMFobs, I=Ki_Iab_EMFobs}
      mask prompts: Rs "Resistance"; Ld "Inductance"; P "Simulink:masks:ProportionalP_MP"; I "Simulink:masks:IntegralI_MP"
      mask TypeOptions Rs: DC Motor Model/Resistance/Gain
      mask TypeOptions Ld: DC Motor Model/Inductance/Gain
      mask TypeOptions P: PID Controller/P
      mask TypeOptions I: PID Controller/I
      mask DialogControl Container6 Prompt: PI Controller
      mask DialogControl P Prompt: Proportional (P):
      mask DialogControl I Prompt: Integral (I):
  EMF Observer Ia2 : Subsystem  mask{Rs=EMFobsRS, Ld=EMFobsLdGain, P=Kp_Iab_EMFobs, I=Ki_Iab_EMFobs}
      mask prompts: Rs "Resistance"; Ld "Inductance"; P "Simulink:masks:ProportionalP_MP"; I "Simulink:masks:IntegralI_MP"
      mask TypeOptions Rs: DC Motor Model/Resistance/Gain
      mask TypeOptions Ld: DC Motor Model/Inductance/Gain
      mask TypeOptions P: PID Controller/P
      mask TypeOptions I: PID Controller/I
      mask DialogControl Container6 Prompt: PI Controller
      mask DialogControl P Prompt: Proportional (P):
      mask DialogControl I Prompt: Integral (I):
  Low pass filter : Subsystem  mask{Value=CuttOffFreq_c, Gain=250e-6}
      mask prompts: Value "CuttOff Freq."; Gain "Time interval"
      settings: AttributesFormatString=Integration constant %<Gain>
      mask TypeOptions Value: Constant/Value
      mask TypeOptions Gain: Gain/Gain
  Low pass filter1 : Subsystem  mask{Value=CuttOffFreq_c, Gain=250e-6}
      mask prompts: Value "CuttOff Freq."; Gain "Time interval"
      settings: AttributesFormatString=Integration constant %<Gain>
      mask TypeOptions Value: Constant/Value
      mask TypeOptions Gain: Gain/Gain
  Low pass filter2 : Subsystem  mask{Value=CuttOffFreq_c, Gain=250e-6}
      mask prompts: Value "CuttOff Freq."; Gain "Time interval"
      settings: AttributesFormatString=Integration constant %<Gain>
      mask TypeOptions Value: Constant/Value
      mask TypeOptions Gain: Gain/Gain
  Low pass filter3 : Subsystem  mask{Value=CuttOffFreq_c, Gain=250e-6}
      mask prompts: Value "CuttOff Freq."; Gain "Time interval"
      settings: AttributesFormatString=Integration constant %<Gain>
      mask TypeOptions Value: Constant/Value
      mask TypeOptions Gain: Gain/Gain
  Unit Delay : UnitDelay  SampleTime=-1  HasFrameUpgradeWarning=on
  Unit Delay1 : UnitDelay  SampleTime=-1  HasFrameUpgradeWarning=on
  theta : Outport
  wires:
  Atan2/1(Out1) -> theta/1  "theta"
  Va/1 -> EMF Observer Ia/2(Vab)
  Ia/1 -> EMF Observer Ia/1(Iab)  "Ia measured"
  Vb/1 -> EMF Observer Ia2/2(Vab)
  Ib/1 -> EMF Observer Ia2/1(Iab)
  EMF Observer Ia/1(BackEMFest) -> Low pass filter/1(In1)
  Low pass filter/1(Output) -> Low pass filter1/1(In1), Unit Delay/1  "Sig_First_LPF_out"
  EMF Observer Ia2/1(BackEMFest) -> Low pass filter3/1(In1)
  Low pass filter3/1(Output) -> Low pass filter2/1(In1), Unit Delay1/1
  Low pass filter1/1(Output) -> Atan2/1(In1)  "Sig_Second_LPF_out"
  Low pass filter2/1(Output) -> Atan2/2(In2)
  Unit Delay/1 -> EMF Observer Ia/3(filtered emf)
  Unit Delay1/1 -> EMF Observer Ia2/3(filtered emf)
  In5/1 -> EMF Observer Ia/4(reset), EMF Observer Ia2/4(reset)

== system MotorControlLibNEWFixedP_FULL/Start up ==
  In1 : Inport
  In2 : Inport  Port=2
  Logic after motor is stoped : Subsystem
  Simulate start up Theta : Subsystem
  theta : Outport
  logic : Outport  Port=2
  wires:
  In1/1 -> Logic after motor is stoped/1(In1)
  Logic after motor is stoped/1(Out1) -> logic/1
  In2/1 -> Simulate start up Theta/1(In1)
  Simulate start up Theta/1(Out1) -> theta/1

== system MotorControlLibNEWFixedP_FULL/Commented/Subsystem ==
  Clock : Inport
  function : TriggerPort  TriggerType=function-call  VariantControl=Variant
  Add2 : Sum  Inputs=+-
  Unit Conversion1 : UnitConversion  OutputType=Inherit: Inherit via back propagation
  Unit Delay : UnitDelay  SampleTime=-1  HasFrameUpgradeWarning=on
  dt : Outport
  wires:
  Add2/1 -> Unit Conversion1/1  "TimeMS"
  Unit Delay/1 -> Add2/2
  Clock/1 -> Unit Delay/1, Add2/1
  Unit Conversion1/1 -> dt/1  "Tsec"

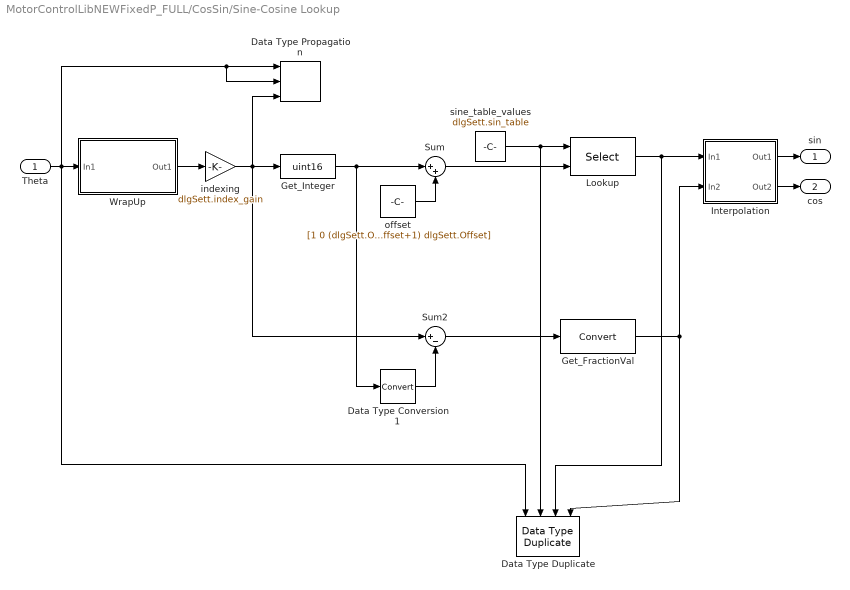
== system MotorControlLibNEWFixedP_FULL/CosSin/Sine-Cosine Lookup ==
  Theta : Inport
  Data Type Duplicate : DataTypeDuplicate  NumInputPorts=4
  Data Type Propagation : simulink/Signal Attributes/Data Type Propagation  PropDataType=fixdt(1, 16)  IfRefDouble=double  IfRefSingle=single  IsSigned=IsSigned1 or IsSigned2  NumBitsBase=max([NumBits1 NumBits2])  NumBitsMult=1  NumBitsAdd=0  NumBitsAllowFinal=1:128  PropScalingMode=Obtain via best precision  PropScaling=2^-10  ValuesUsedBestPrec=[0 dlgSett.index_gain]  SlopeBase=min([Slope1 Slope2])  SlopeMult=1  SlopeAdd=0  BiasBase=Bias1  BiasMult=1  BiasAdd=0
      settings: SourceProductBaseCode=SL
  Data Type Conversion1 : DataTypeConversion  RndMeth=Simplest
  Get_FractionVal : DataTypeConversion  RndMeth=Simplest
  Get_Integer : DataTypeConversion  OutDataTypeStr=uint16  RndMeth=Simplest
  Interpolation : Subsystem
  Lookup : Selector  IndexMode=Zero-based  InputPortWidth=dlgSett.size  IndexOptions=Index vector (port)  Indices=[1 3]  OutputSizes=1
  Sum : Sum  Inputs=|++  AccumDataTypeStr=uint32  OutDataTypeStr=uint32  RndMeth=Simplest
  Sum2 : Sum  Inputs=|+-  RndMeth=Simplest  OutDataTypeStr=Inherit: Same as first input
  WrapUp : Subsystem
  indexing : Gain  Gain=dlgSett.index_gain  OutDataTypeStr=Inherit: Inherit via back propagation  RndMeth=Simplest
  offset : Constant  Value=[1 0 (dlgSett.Offset+1) dlgSett.Offset]  OutDataTypeStr=int16  SampleTime=-1
  sine_table_values : Constant  Value=dlgSett.sin_table  OutDataTypeStr=Inherit: Inherit via back propagation  SampleTime=-1
  sin : Outport  VectorParamsAs1DForOutWhenUnconnected=off
  cos : Outport  Port=2  VectorParamsAs1DForOutWhenUnconnected=off
  wires:
  Interpolation/2(Out2) -> cos/1
  Interpolation/1(Out1) -> sin/1
  Sum/1 -> Lookup/2
  indexing/1 -> Sum2/1, Data Type Propagation/3, Get_Integer/1
  Data Type Conversion1/1 -> Sum2/2
  Get_Integer/1 -> Sum/1, Data Type Conversion1/1
  offset/1 -> Sum/2
  sine_table_values/1 -> Lookup/1, Data Type Duplicate/2
  Lookup/1 -> Interpolation/1(In1), Data Type Duplicate/3
  Sum2/1 -> Get_FractionVal/1
  Get_FractionVal/1 -> Data Type Duplicate/4, Interpolation/2(In2)
  Theta/1 -> Data Type Duplicate/1, WrapUp/1(In1), Data Type Propagation/2, Data Type Propagation/1
  WrapUp/1(Out1) -> indexing/1

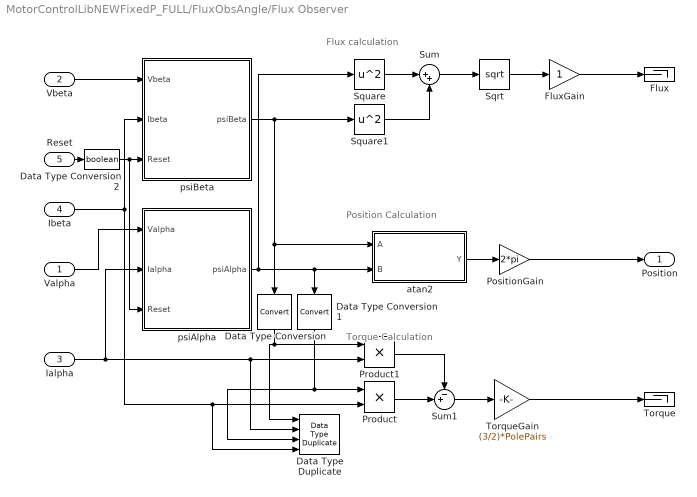
== system MotorControlLibNEWFixedP_FULL/FluxObsAngle/Flux Observer ==
  note: Torque Calculation
  note: Position Calculation
  note: Flux calculation
  Valpha : Inport  SampleTime=BlockSampleTime
  Vbeta : Inport  Port=2  SampleTime=BlockSampleTime
  Ialpha : Inport  Port=3  SampleTime=BlockSampleTime
  Ibeta : Inport  Port=4  SampleTime=BlockSampleTime
  Reset : Inport  Port=5  SampleTime=BlockSampleTime
  Data Type Duplicate : DataTypeDuplicate  NumInputPorts=4
  Data Type Conversion : DataTypeConversion  RndMeth=Simplest
  Data Type Conversion1 : DataTypeConversion  RndMeth=Simplest
  Data Type Conversion2 : DataTypeConversion  OutDataTypeStr=boolean  RndMeth=Simplest
  Flux : Terminator
  FluxGain : Gain  OutDataTypeStr=FluxDatatype  RndMeth=Simplest
  PositionGain : Gain  Gain=2*pi  OutDataTypeStr=PositionDatatype  RndMeth=Simplest
  Product : Product  RndMeth=Simplest  OutDataTypeStr=Inherit: Same as first input
  Product1 : Product  RndMeth=Simplest  OutDataTypeStr=Inherit: Same as first input
  Sqrt : Sqrt  RndMeth=Simplest  IntermediateResultsDataTypeStr=Inherit: Inherit from input  SaturateOnIntegerOverflow=on
  Square : Math  Operator=square  RndMeth=Simplest  SaturateOnIntegerOverflow=on
  Square1 : Math  Operator=square  RndMeth=Simplest  SaturateOnIntegerOverflow=on
  Sum : Sum  Inputs=|++
  Sum1 : Sum  Inputs=-+|
  Torque : Terminator
  TorqueGain : Gain  Gain=(3/2)*PolePairs  OutDataTypeStr=TorqueDatatype
  atan2 : Subsystem  TreatAsAtomicUnit=on  mask(atan2){outputUnit=PerUnit}
      mask prompts: outputUnit "Output unit:"
      mask help:
      | Compute the four-quadrant arctangent for two real numbers.
      |
      | The output datatype is identical to the inputs.
      |
      | The block output ranges from -pi to +pi (Radians) or 0 to 1 (PerUnit).
      mask Help: eval('mcb.internal.helpview(''atantwo'')')
      mask TypeOptions outputUnit: Radians | PerUnit
      mask Callback outputUnit: set_param([gcb, '/a16'],'AlgorithmParameterValue1',get_param(gcb,'outputUnit'))
      mask DialogControl Container7 Prompt: Parameters
      mask Display:
      | color('black');
      | port_label('input',1, 'A');
      | port_label('input',2, 'B');,
      | port_label('output',1, '\theta', 'interpreter', 'tex');
      | fprintf('atan2');
  psiAlpha : Subsystem
  psiBeta : Subsystem
  Position : Outport
  wires:
  Valpha/1 -> psiAlpha/1(Valpha)
  Ibeta/1 -> psiBeta/2(Ibeta), Data Type Duplicate/4, Product/2
  Vbeta/1 -> psiBeta/1(Vbeta)
  Reset/1 -> Data Type Conversion2/1
  TorqueGain/1 -> Torque/1
  Product/1 -> Sum1/2
  psiBeta/1(psiBeta) -> Square1/1, atan2/1(A), Data Type Conversion/1
  psiAlpha/1(psiAlpha) -> atan2/2(B), Data Type Conversion1/1, Square/1
  Ialpha/1 -> psiAlpha/2(Ialpha), Data Type Duplicate/2, Product1/2
  Product1/1 -> Sum1/1
  Sum1/1 -> TorqueGain/1
  FluxGain/1 -> Flux/1
  Square/1 -> Sum/1
  Sum/1 -> Sqrt/1
  Square1/1 -> Sum/2
  Sqrt/1 -> FluxGain/1
  PositionGain/1 -> Position/1
  atan2/1(Y) -> PositionGain/1
  Data Type Conversion/1 -> Data Type Duplicate/1, Product1/1
  Data Type Conversion1/1 -> Data Type Duplicate/3, Product/1
  Data Type Conversion2/1 -> psiAlpha/3(Reset), psiBeta/3(Reset)

== system MotorControlLibNEWFixedP_FULL/Inverse Park Transform/Switch_Axis ==
  A : Inport
  B : Inport  Port=2
  D_axis_aligned : Mux  Inputs=2
  Demux : Demux  Outputs=2
  Offset : Constant  Value=0  OutDataTypeStr=uint16  SampleTime=-1
  Q_axis_aligned : Mux  Inputs=2
  Switch : Switch  Criteria=u2 > Threshold  Threshold=1  RndMeth=Simplest  ZeroCross=off
  Unary_Minus : UnaryMinus
  Alpha : Outport  VectorParamsAs1DForOutWhenUnconnected=off
  Beta : Outport  Port=2  VectorParamsAs1DForOutWhenUnconnected=off
  wires:
  A/1 -> D_axis_aligned/1, Unary_Minus/1
  Unary_Minus/1 -> Q_axis_aligned/2
  Demux/2 -> Beta/1
  Switch/1 -> Demux/1
  B/1 -> D_axis_aligned/2, Q_axis_aligned/1
  Demux/1 -> Alpha/1
  Offset/1 -> Switch/2
  Q_axis_aligned/1 -> Switch/1
  D_axis_aligned/1 -> Switch/3

== system MotorControlLibNEWFixedP_FULL/PWM Output/Inverse Clarke Transform ==
  In1 : Inport
  In2 : Inport  Port=2
  Data Type Duplicate : DataTypeDuplicate
  add_b : Sum  Inputs=-+  RndMeth=Simplest  OutDataTypeStr=Inherit: Same as first input
  add_c : Sum  Inputs=--  RndMeth=Simplest  OutDataTypeStr=Inherit: Same as first input
  one_by_two : Gain  Gain=1/2  RndMeth=Simplest  OutDataTypeStr=Inherit: Same as input
  sqrt3_by_two : Gain  Gain=sqrt(3)/2  RndMeth=Simplest  OutDataTypeStr=Inherit: Same as input
  a : Outport  VectorParamsAs1DForOutWhenUnconnected=off
  b : Outport  Port=2  VectorParamsAs1DForOutWhenUnconnected=off
  c : Outport  Port=3  VectorParamsAs1DForOutWhenUnconnected=off
  wires:
  add_c/1 -> c/1
  sqrt3_by_two/1 -> add_c/2, add_b/2
  In1/1 -> one_by_two/1, Data Type Duplicate/1, a/1
  one_by_two/1 -> add_b/1, add_c/1
  In2/1 -> sqrt3_by_two/1, Data Type Duplicate/2
  add_b/1 -> b/1

== system MotorControlLibNEWFixedP_FULL/Park Transform/Switch_Axis ==
  d : Inport
  q : Inport  Port=2
  D_axis_aligned : Mux  Inputs=2
  Demux : Demux  Outputs=2
  Offset : Constant  Value=0  OutDataTypeStr=uint16  SampleTime=-1
  Q_axis_aligned : Mux  Inputs=2
  Switch : Switch  Criteria=u2 > Threshold  Threshold=1  RndMeth=Simplest  ZeroCross=off
  Unary_Minus : UnaryMinus
  d_axis : Outport  VectorParamsAs1DForOutWhenUnconnected=off
  q_axis : Outport  Port=2  VectorParamsAs1DForOutWhenUnconnected=off
  wires:
  D_axis_aligned/1 -> Switch/3
  Q_axis_aligned/1 -> Switch/1
  d/1 -> D_axis_aligned/1, Q_axis_aligned/2
  Offset/1 -> Switch/2
  Demux/1 -> d_axis/1
  Unary_Minus/1 -> Q_axis_aligned/1
  q/1 -> D_axis_aligned/2, Unary_Minus/1
  Switch/1 -> Demux/1
  Demux/2 -> q_axis/1

== system MotorControlLibNEWFixedP_FULL/Position observer/Atan2 ==
  In1 : Inport
  In2 : Inport  Port=2
  Atan2 : Trigonometry  Operator=atan2  ApproximationMethod=CORDIC  NumberOfIterations=6
  Data Type Conversion5 : DataTypeConversion
  Data Type Conversion6 : DataTypeConversion  OutDataTypeStr=single
  Data Type Conversion7 : DataTypeConversion  OutDataTypeStr=single
  Out1 : Outport
  wires:
  Atan2/1 -> Data Type Conversion5/1
  In1/1 -> Data Type Conversion6/1
  Data Type Conversion6/1 -> Atan2/1
  Data Type Conversion7/1 -> Atan2/2
  In2/1 -> Data Type Conversion7/1
  Data Type Conversion5/1 -> Out1/1

== system MotorControlLibNEWFixedP_FULL/Position observer/EMF Observer Ia ==
  Iab : Inport
  Vab : Inport  Port=2
  filtered emf : Inport  Port=3
  reset : Inport  Port=4
  Add6 : Sum  Inputs=-+  InputSameDT=on
  DC Motor Model : Subsystem  TreatAsAtomicUnit=on  SystemSampleTime=Ts
  PI Controller : Subsystem
  Rate Transition{,1..3} (4 alike) : RateTransition  Integrity=off
  Unit Delay : UnitDelay  SampleTime=-1  HasFrameUpgradeWarning=on
  BackEMFest : Outport
  wires:
  Iab/1 -> Add6/1
  DC Motor Model/1(i_integrated_en8) -> Rate Transition/1
  Vab/1 -> Rate Transition1/1
  Rate Transition/1 -> Add6/2  "Iest"
  Rate Transition1/1 -> DC Motor Model/2(In2)
  Rate Transition2/1 -> DC Motor Model/1(Sig_Emfobs_PI_out)
  PI Controller/1(Sig_Emfobs_PI_out) -> Unit Delay/1, BackEMFest/1  "BackEMF est"
  Add6/1 -> PI Controller/1(Sig_Emfobs_errorSum_m)  "Sig_Emfobs_errorSum_m"
  filtered emf/1 -> Rate Transition3/1
  Rate Transition3/1 -> DC Motor Model/3(In3)
  Unit Delay/1 -> Rate Transition2/1
  reset/1 -> PI Controller/2(reset)

== system MotorControlLibNEWFixedP_FULL/Position observer/EMF Observer Ia1 ==
  Iab : Inport
  Vab : Inport  Port=2
  DC Motor Model : Subsystem
  PI Controller : Subsystem
  Rate Transition : RateTransition
  Rate Transition1 : RateTransition
  Rate Transition2 : RateTransition
  Unit Delay : UnitDelay  SampleTime=-1  HasFrameUpgradeWarning=on
  Iestimated : Outport
  IestNEW : Outport  Port=2
  wires:
  DC Motor Model/1(Out1) -> Rate Transition/1
  Vab/1 -> Rate Transition1/1
  Rate Transition/1 -> PI Controller/2(In2), IestNEW/1
  Rate Transition1/1 -> DC Motor Model/2(In2)
  Rate Transition2/1 -> DC Motor Model/1(In1)
  PI Controller/1(Out1) -> Iestimated/1, Unit Delay/1
  Iab/1 -> PI Controller/1(In1)
  Unit Delay/1 -> Rate Transition2/1

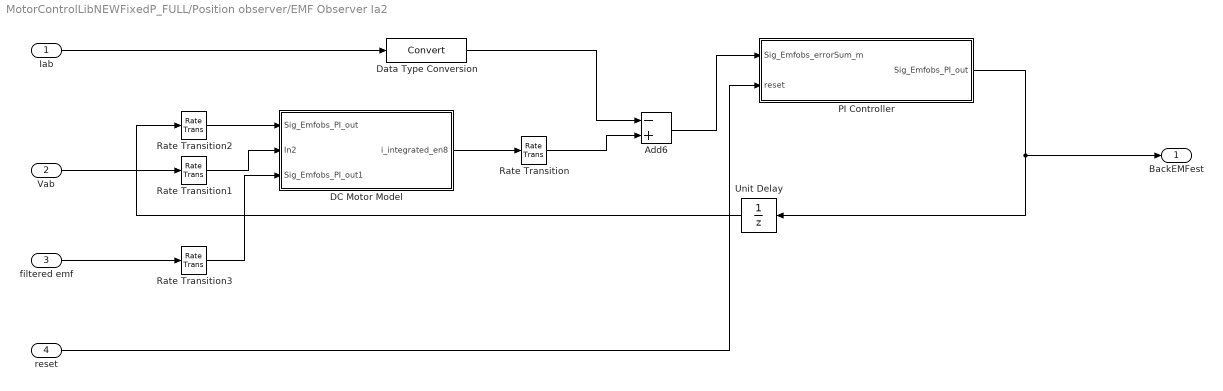
== system MotorControlLibNEWFixedP_FULL/Position observer/EMF Observer Ia2 ==
  Iab : Inport
  Vab : Inport  Port=2
  filtered emf : Inport  Port=3
  reset : Inport  Port=4
  Add6 : Sum  Inputs=-+  InputSameDT=on
  DC Motor Model : Subsystem  TreatAsAtomicUnit=on  SystemSampleTime=Ts
  Data Type Conversion : DataTypeConversion
  PI Controller : Subsystem  TreatAsAtomicUnit=on
  Rate Transition{,1..3} (4 alike) : RateTransition  Integrity=off
  Unit Delay : UnitDelay  SampleTime=-1  HasFrameUpgradeWarning=on
  BackEMFest : Outport
  wires:
  PI Controller/1(Sig_Emfobs_PI_out) -> Unit Delay/1, BackEMFest/1
  Add6/1 -> PI Controller/1(Sig_Emfobs_errorSum_m)
  Rate Transition2/1 -> DC Motor Model/1(Sig_Emfobs_PI_out)
  Rate Transition1/1 -> DC Motor Model/2(In2)
  Rate Transition/1 -> Add6/2
  Vab/1 -> Rate Transition1/1
  DC Motor Model/1(i_integrated_en8) -> Rate Transition/1
  Iab/1 -> Data Type Conversion/1
  Data Type Conversion/1 -> Add6/1
  filtered emf/1 -> Rate Transition3/1
  Rate Transition3/1 -> DC Motor Model/3(Sig_Emfobs_PI_out1)
  Unit Delay/1 -> Rate Transition2/1
  reset/1 -> PI Controller/2(reset)

== system MotorControlLibNEWFixedP_FULL/Position observer/Low pass filter ==
  note: Integrator
  note: d/dt(i)
  In1 : Inport
  Add2 : Sum  Inputs=+-
  Constant : Constant  Value=Value  OutDataTypeStr=uint16
  Delay : Delay  DelayLength=1  InitialCondition=0
  Gain : Gain  Gain=Gain  ParamDataTypeStr=fixdt(1,16,2^-16,0)  OutDataTypeStr=fixdt(1,16,2^-14,0)  SaturateOnIntegerOverflow=on
  Product1 : Product  OutDataTypeStr=fixdt(1,16,2^-6,0)
  Sum : Sum  Inputs=|++  OutDataTypeStr=Inherit: Same as first input
  Unit Delay : UnitDelay  SampleTime=-1  HasFrameUpgradeWarning=on
  Output : Outport
  wires:
  Constant/1 -> Product1/2
  In1/1 -> Add2/1
  Add2/1 -> Gain/1
  Product1/1 -> Output/1, Unit Delay/1
  Gain/1 -> Sum/1
  Delay/1 -> Sum/2
  Sum/1 -> Delay/1, Product1/1
  Unit Delay/1 -> Add2/2
